simulink model "Simulacion_5_1_2_D"  (R2020a)
settings: Solver=ode45  StartTime=0.0  StopTime=10.0  MaxStep=1e-4  RelTol=1e-3
values from neighbouring files (symbols this model uses):
  A = [ 0        1               0 ... (first row only)    [AnalisisDeEstabilidad.m]    (also in Consigna_de_pos.m = [t_1^3,t_1^2,t_1,1; Controlabilidad.m = [0 ,       1      ,         0; Funciones_de_Transferencia.m = [ 0         1                           0; LTI_vs_LPV_vs_NL_realimentado.m = [0                                                       1  )
  B = [0              0 ... (first row only)    [AnalisisDeEstabilidad.m]    (also in Consigna_de_pos.m = [theta_m1; theta_m2; 0 ;0]; Controlabilidad.m = [0;0;1/Lq]; LTI_vs_LPV_vs_NL_realimentado.m = [0      0       0           0           0; Modelo_linealizado.m = [0,0,0,0,0)
  b_eq = b_m + b_l/(r^2)    (= 2.19444444444e-05)    [LTI_vs_LPV_vs_NL_realimentado.m]    (also in Modelo_linealizado.m; parametros.m)
  C = [1 0 0]    [AnalisisDeEstabilidad.m]    (also in LTI_vs_LPV_vs_NL_realimentado.m = eye(6); Modelo_linealizado.m = eye(6); Obsevabilidad.m = [1,0,0,0,0])
  C_ts = 0.818    [LTI_vs_LPV_vs_NL_realimentado.m]    (also in Modelo_linealizado.m; parametros.m)
  D = [0 0]    [AnalisisDeEstabilidad.m]    (also in LTI_vs_LPV_vs_NL_realimentado.m = zeros(6,5); Modelo_linealizado.m = zeros(6,5))
  J_eq = J_m + J_l/(r^2)    (= 1.97847222222e-05)    [LTI_vs_LPV_vs_NL_realimentado.m]    (also in Modelo_linealizado.m; parametros.m)
  L_d = 6.6/1000    (= 0.0066)    [Curvas_carc.m]    (also in LTI_vs_LPV_vs_NL_realimentado.m; Modelo_linealizado.m; parametros.m)
  L_ls = 0.8/1000    (= 0.0008)    [LTI_vs_LPV_vs_NL_realimentado.m]    (also in Modelo_linealizado.m; parametros.m)
  L_q = 5.8/1000    (= 0.0058)    [Curvas_carc.m]    (also in LTI_vs_LPV_vs_NL_realimentado.m; Modelo_linealizado.m; parametros.m)
  lambda_m = 0.01546    [Curvas_carc.m]    (also in LTI_vs_LPV_vs_NL_realimentado.m = 0.016; Modelo_linealizado.m = 0.016; parametros.m)
  omega_m = linspace(0,100,100)    [Curvas_carc.m]    (also in LTI_vs_LPV_vs_NL_realimentado.m = 0; Modelo_linealizado.m = 0)
  P_p = 3    [Curvas_carc.m]    (also in LTI_vs_LPV_vs_NL_realimentado.m; parametros.m)
  r = 120    [AnalisisDeEstabilidad.m]    (also in LTI_vs_LPV_vs_NL_realimentado.m; Modelo_linealizado.m; parametros.m)
  R_s = 1.02    [Curvas_carc.m]    (also in LTI_vs_LPV_vs_NL_realimentado.m = R_s_o; Modelo_linealizado.m = 0.348)
  R_ts_amb = 146.7    [LTI_vs_LPV_vs_NL_realimentado.m]    (also in Modelo_linealizado.m; parametros.m)
  theta_m = pi/3    (= 1.0471975512)    [LTI_vs_LPV_vs_NL_realimentado.m]    (also in Modelo_linealizado.m)
undefined symbols (not defined in the file or in its folder): i_ds, i_os, i_qs, K_l, T_s
settings Model: Creator=matie  LastModifiedBy=Juan

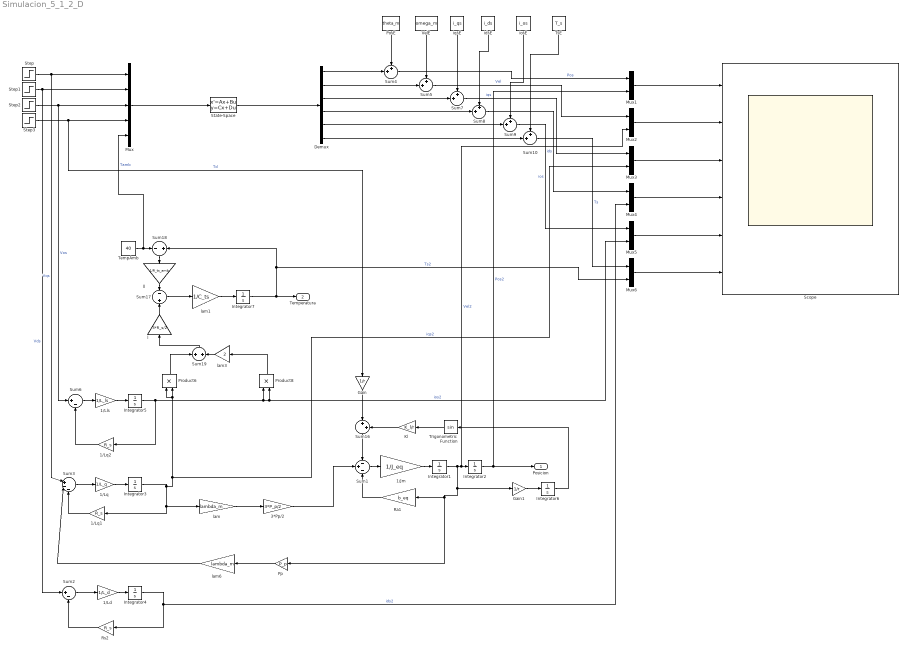
== system Simulacion_5_1_2_D ==
  1/Jm : Gain  Gain=1/J_eq
  1/Ld : Gain  Gain=1/L_d
  1/Lls : Gain  Gain=1/L_ls
  1/Lq : Gain  Gain=1/L_q
  1/Lq1 : Gain  Gain=R_s
  1/Lq2 : Gain  Gain=R_s
  3*Pp/2 : Gain  Gain=3*P_p/2
  Demux : Demux  Outputs=6
  Gain : Gain  Gain=1/r
  Gain1 : Gain  Gain=1/r
  Integrator{1..7} (7 alike) : Integrator
  Kl : Gain  Gain=K_l/r
  Mux : Mux  Inputs=5
  Mux{1..6} (6 alike) : Mux  Inputs=2
  PosE : Constant  Value=theta_m
  Pp : Gain  Gain=P_p
  Product6 : Product
  Product8 : Product
  Ra1 : Gain  Gain=b_eq
  Rs2 : Gain  Gain=R_s
  Scope : Scope  NumInputPorts=6
  State-Space : StateSpace  A=A  B=B  C=C  D=D  InitialCondition=0
  Step : Step  After=0.01  SampleTime=0
  Step1 : Step  Time=0  After=0  SampleTime=0
  Step2 : Step  Time=0  After=0  SampleTime=0
  Step3 : Step  Time=0  After=0  SampleTime=0
  Sum1 : Sum  Inputs=-+-
  Sum{4..5,7..10} (6 alike) : Sum  Inputs=++|
  Sum16 : Sum  Inputs=|++
  Sum17 : Sum  Inputs=-+
  Sum18 : Sum  Inputs=-+
  Sum19 : Sum
  Sum2 : Sum  Inputs=|+-
  Sum3 : Sum  Inputs=|+--
  Sum6 : Sum  Inputs=|+-
  TempAmb : Constant  Value=40
  Trigonometric Function : Trigonometry
  TsE : Constant  Value=T_s
  VelE : Constant  Value=omega_m
  idsE : Constant  Value=i_ds
  iosE : Constant  Value=i_os
  iqsE : Constant  Value=i_qs
  l : Gain  Gain=3*R_s/2
  lam : Gain  Gain=lambda_m
  lam1 : Gain  Gain=1/C_ts
  lam3 : Gain  Gain=2
  lam6 : Gain  Gain=lambda_m
  ll : Gain  Gain=1/R_ts_amb
  Posicion : Outport
  Temperatura : Outport  Port=2
  wires:
  State-Space/1 -> Demux/1
  Demux/1 -> Sum4/2
  Demux/2 -> Sum5/2
  Demux/3 -> Sum7/2
  Demux/4 -> Sum8/2
  Demux/5 -> Sum9/2
  Demux/6 -> Sum10/2
  Mux/1 -> State-Space/1
  Step/1 -> Sum3/1, Mux/1  "Vqs"
  Step2/1 -> Mux/3, Sum6/1  "Vos"
  Step3/1 -> Gain/1, Mux/4  "Td"
  TempAmb/1 -> Mux/5, Sum18/1  "Tamb"
  Sum19/1 -> l/1
  Sum3/1 -> 1/Lq/1
  Pp/1 -> lam6/1
  Sum1/1 -> 1/Jm/1
  1/Ld/1 -> Integrator4/1
  1/Jm/1 -> Integrator1/1
  l/1 -> Sum17/2
  lam/1 -> 3*Pp/2/1
  Integrator4/1 -> Mux4/2, Rs2/1  "ids2"
  lam1/1 -> Integrator7/1
  Integrator2/1 -> Posicion/1, Mux1/2  "Pos2"
  Integrator3/1 -> 1/Lq1/1, lam/1, Mux3/2, Product6/1, Product6/2  "iqs2"
  Sum17/1 -> lam1/1
  Ra1/1 -> Sum1/3
  1/Lq/1 -> Integrator3/1
  Trigonometric Function/1 -> Kl/1
  Product8/1 -> lam3/1
  1/Lq1/1 -> Sum3/3
  3*Pp/2/1 -> Sum1/2
  1/Lq2/1 -> Sum6/2
  Integrator6/1 -> Trigonometric Function/1
  ll/1 -> Sum17/1
  Sum16/1 -> Sum1/1
  Gain/1 -> Sum16/1
  Product6/1 -> Sum19/1
  lam6/1 -> Sum3/2
  Integrator7/1 -> Sum18/2, Mux6/2, Temperatura/1  "Ts2"
  Sum18/1 -> ll/1
  Integrator5/1 -> 1/Lq2/1, Mux5/2, Product8/2, Product8/1  "ios2"
  lam3/1 -> Sum19/2
  Sum6/1 -> 1/Lls/1
  Kl/1 -> Sum16/2
  Integrator1/1 -> Gain1/1, Pp/1, Ra1/1, Mux2/2, Integrator2/1  "Vel2"
  Gain1/1 -> Integrator6/1
  1/Lls/1 -> Integrator5/1
  Rs2/1 -> Sum2/2
  Sum2/1 -> 1/Ld/1
  Step1/1 -> Mux/2, Sum2/1  "Vds"
  Mux1/1 -> Scope/1
  Mux2/1 -> Scope/2
  Mux3/1 -> Scope/3
  Mux4/1 -> Scope/4
  Mux5/1 -> Scope/5
  Mux6/1 -> Scope/6
  Sum4/1 -> Mux1/1  "Pos"
  PosE/1 -> Sum4/1
  Sum5/1 -> Mux2/1  "Vel"
  VelE/1 -> Sum5/1
  Sum7/1 -> Mux3/1  "iqs"
  iqsE/1 -> Sum7/1
  Sum8/1 -> Mux4/1  "ids"
  idsE/1 -> Sum8/1
  Sum9/1 -> Mux5/1  "ios"
  iosE/1 -> Sum9/1
  Sum10/1 -> Mux6/1  "Ts"
  TsE/1 -> Sum10/1
